simulink model "Cognata_Amp_Tobi_Split"  (R2020a)
settings: Solver=VariableStepAuto  StartTime=0.0  StopTime=inf  RelTol=1e-3
model workspace (MAT data in the model file):
  WinSize = Simulink.Parameter
  WinSize.Value = 16
  WinSize.DataType = 'double'
  WinSize.Dimensions = [1 1]
  fc_bandpass = Simulink.Parameter
  fc_bandpass.Value = [0.05 0.26]
  fc_bandpass.DataType = 'auto'
  fc_bandpass.Dimensions = [1 2]
undefined symbols (not defined in the file or in its folder): currentCFG_Cognata_Amp_Tobi_split_UB, fdesignblkfcn, gcbh, UB
libraries: gtecHighspeedLib x17, robotlib x12, dspfdesign x3, simulink x2, dsparch4 x2, TobiiEyeTrackerLib x1, gUSBamplib x1
settings Model: Creator=LAB-OREN3  LastModifiedBy=LAB-OREN3

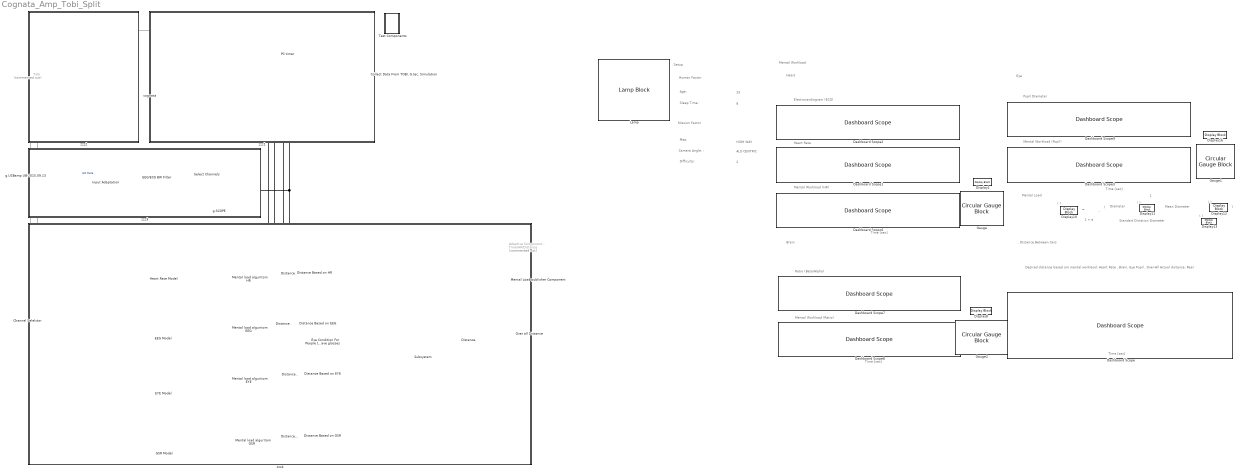
== system Cognata_Amp_Tobi_Split ==
  note: Time [sec]
  note: . Setup
  note: ( )
  note: Desired distance based om mental worklaod:
      | Heart Rate , Brain, Eye Pupil , Over-All
      |
      | Actual distance: Real
  note: Mission Factor
  note: Mental Workload (HR)
  note: Ratio (Beta/Alpha)
  note: 1
  note: Mental Load
  note: ( )
  note: Map:
  note: (
  note: HIGH WAY
  note: Mental Workload (Ratio)
  note: Eye
  note: 25
  note: Mean Diameter
  note: Time [sec]
  note: Diameter
  note: Human Factor
  note: Standart Diviation Diameter
  note: Age:
  note: Difficulty:
  note: 1 + e
  note: Camera Angle: :
  note: 8
  note: Sleep Time:
  note: Electrocardiogram (ECG)
  note: Heart
  note: Time [sec]
  note: ALO CENTRIC
  note: Brain
  note: Heart Rate
  note: ( )
  note: Pupil Diameter
  note: )
  note: -
  note: Mental Workload (Pupil)
  note: . Distance Between Cars
  note: 2
  note: ( )
  note: Time [sec]
  note: =
  note: Mental Workload
  "Adaptive Component - Time/HR/Distance " : Subsystem  Commented=on
  Channel Selelctor : Subsystem
  "Collect Data From TOBI, G.tec, Simulation" : Subsystem
  Dashboard Scope : DashboardScope  ShowInitialText=off  TimeSpan=10  Ymin=-1  Ymax=20  LegendPosition=Hide  ScaleAtStop=off
  Dashboard Scope1 : DashboardScope  TimeSpan=10  Ymin=0  Ymax=100  LegendPosition=Hide  ScaleAtStop=off
  Dashboard Scope2 : DashboardScope  TimeSpan=10  Ymin=-3000  Ymax=1000  LegendPosition=Hide  ScaleAtStop=off
  Dashboard Scope3 : DashboardScope  TimeSpan=10  Ymin=0  Ymax=1  LegendPosition=Hide  ScaleAtStop=off
  Dashboard Scope6 : DashboardScope  TimeSpan=10  Ymin=0  Ymax=1  LegendPosition=Hide  ScaleAtStop=off
  Dashboard Scope7 : DashboardScope  TimeSpan=10  Ymin=0  Ymax=0.5  LegendPosition=Hide  ScaleAtStop=off
  Dashboard Scope8 : DashboardScope  TimeSpan=10  Ymin=0  Ymax=1  LegendPosition=Hide  ScaleAtStop=off
  Dashboard Scope9 : DashboardScope  TimeSpan=10  Ymin=0  Ymax=5  LegendPosition=Hide  ScaleAtStop=off
  Display{1,8,10..11,13,16} (6 alike) : DisplayBlock  LabelPosition=Hide  Format=bank  Transparency=1
  Display12 : DisplayBlock  LabelPosition=Hide  Format=bank  Transparency=1  Layout=Fill available space
  Distance : MATLAB Function  TreatAsAtomicUnit=on
  Distance Based on EEG : Display
  Distance Based on EYE : Display
  Distance Based on GSR : Display
  Distance Based on HR : Display
  Distance, : MATLAB Function  TreatAsAtomicUnit=on
  Distance. : MATLAB Function  TreatAsAtomicUnit=on
  Distance.. : MATLAB Function  TreatAsAtomicUnit=on
  Distance... : MATLAB Function  TreatAsAtomicUnit=on
  EEG Model : Subsystem  ReferencedSubsystem=EEG_Ratio_Model
  EEG/ECG BW Filter : gtecHighspeedLib/EEG//ECG BW Filter  Order=6  LowerFreq=0.1  UpperFreq=30  SampFreq=512
      settings: SourceProductName=g.HIsys Library
  EYE Model : Subsystem  ReferencedSubsystem=Pupil_Diameter_Model
  Eye Condition For People that have glasses : Constant  Value=0
  GSR Model : Subsystem  ReferencedSubsystem=GSR_Model
  Gauge : CircularGaugeBlock  LabelPosition=Hide  ScaleMax=1  TickInterval=0.2
  Gauge1 : CircularGaugeBlock  LabelPosition=Hide  ScaleMax=1  TickInterval=0.2
  Gauge2 : CircularGaugeBlock  LabelPosition=Hide  ScaleMax=1  TickInterval=0.2
  Heart Rate Model : Subsystem  ReferencedSubsystem=Heart_Rate_Model
  Input Adaptation : Subsystem
  Lamp : LampBlock
  Mental Load publisher Component : Subsystem
  "Mental load alguritom EEG " : MATLAB Function  TreatAsAtomicUnit=on
  Mental load alguritom EYE : MATLAB Function  TreatAsAtomicUnit=on
  Mental load alguritom GSR : MATLAB Function  TreatAsAtomicUnit=on
  Mental load alguritom HR : MATLAB Function  TreatAsAtomicUnit=on
  Over all Distance : Display
  PC timer : MATLAB Function  TreatAsAtomicUnit=on
  Select Channels : gtecHighspeedLib/Select Channels  selectedchannels=[2]  totalchannels=14
      settings: SourceProductName=g.HIsys Library
  Subsystem : Subsystem
  Test Components : Subsystem
  Tobi : Subsystem  Commented=on
  cognata : Subsystem
  g.SCOPE : gtecHighspeedLib/g.SCOPE
      settings: SourceProductName=g.HIsys Library
  g.USBamp UB-2015.09.13 : gUSBamplib/g.USBamp  cfg=currentCFG_Cognata_Amp_Tobi_split_UB-2015.09.13.cfg  snr=UB-2015.09.13
      settings: SourceProductName=g.USBamp
  zzz1 : Subsystem  TreatAsAtomicUnit=on
      settings: OpenFcn=% no-op
      mask Display: disp('')
  zzz2 : Subsystem  TreatAsAtomicUnit=on
      settings: OpenFcn=% no-op
      mask Display: disp('')
  zzz3 : Subsystem  TreatAsAtomicUnit=on
      settings: OpenFcn=% no-op
      mask Display: disp('')
  zzz4 : Subsystem  TreatAsAtomicUnit=on
      settings: OpenFcn=% no-op
      mask Display: disp('')
  wires:
  cognata/3(Latitude) -> "Collect Data From TOBI, G.tec, Simulation"/6(Lat), "Adaptive Component - Time/HR/Distance "/3(Lat)
  Distance/1(y) -> Distance Based on HR/1
  EEG Model/1 -> "Mental load alguritom EEG "/1(u)
  Distance../1(y) -> Distance Based on EYE/1
  EYE Model/1 -> Mental load alguritom EYE/1(u)
  Distance,/1(y) -> Over all Distance/1
  g.USBamp UB-2015.09.13/1 -> Input Adaptation/1(In)  "EG Data"
  Mental load alguritom EYE/1(y) -> Distance../1(u), Subsystem/4(eye)
  Mental load alguritom HR/1(y) -> Subsystem/1(HR), Distance/1(u)
  Input Adaptation/1(All channels) -> Channel Selelctor/1(14x1 vec), "Collect Data From TOBI, G.tec, Simulation"/3(G.tec Channels), EEG/ECG BW Filter/1
  Distance./1(y) -> Distance Based on EEG/1
  Select Channels/1 -> ?
  cognata/4(TTC) -> "Collect Data From TOBI, G.tec, Simulation"/7(Distance)
  cognata/1(SimulationTime) -> "Adaptive Component - Time/HR/Distance "/1(Simlulation time), "Collect Data From TOBI, G.tec, Simulation"/4(Simulator time)
  EEG/ECG BW Filter/1 -> g.SCOPE/1, Select Channels/1
  cognata/2(Longitude) -> "Adaptive Component - Time/HR/Distance "/4(Long), "Collect Data From TOBI, G.tec, Simulation"/5(Long)
  "Mental load alguritom EEG "/1(y) -> Subsystem/2(Ratio), Distance./1(u)
  Heart Rate Model/2 -> Mental load alguritom HR/1(u)
  Tobi/1(Sum) -> "Collect Data From TOBI, G.tec, Simulation"/1(Tobi data)
  Mental load alguritom GSR/1(y) -> Distance.../1(u), Subsystem/5(GSR)
  GSR Model/1 -> Mental load alguritom GSR/1(u)
  Distance.../1(y) -> Distance Based on GSR/1
  Tobi/2(Pupil diameter Right) -> EYE Model/2
  Tobi/3("Pupil diameter Left ") -> EYE Model/1
  Subsystem/1(Avrage Mental Load) -> Distance,/1(u), "Adaptive Component - Time/HR/Distance "/2(Avrage Menta Load), Mental Load publisher Component/1(Mental Load)
  Eye Condition For People that have glasses/1 -> Subsystem/3(EyeCondition)
  Channel Selelctor/1(ECG) -> Heart Rate Model/1
  Channel Selelctor/2(EEG1) -> EEG Model/2
  Channel Selelctor/3(EEG2) -> EEG Model/3
  Channel Selelctor/4(EEG3) -> EEG Model/4
  Channel Selelctor/5(EEG4) -> EEG Model/5
  Channel Selelctor/6(EEG5) -> EEG Model/6
  Channel Selelctor/7(EEG6) -> EEG Model/7
  Channel Selelctor/8(EEG7) -> EEG Model/8
  Channel Selelctor/9(EEG8) -> EEG Model/9
  Channel Selelctor/10(EEG9) -> EEG Model/10
  Channel Selelctor/11(EEG10) -> EEG Model/11
  Channel Selelctor/12(EEG11) -> EEG Model/1
  Channel Selelctor/13(GSR) -> GSR Model/1
  PC timer/1(z) -> "Collect Data From TOBI, G.tec, Simulation"/2(PC timer)
  EYE Model/3 -> ?
  EYE Model/2 -> ?
  Channel Selelctor/14(EEG12) -> EEG Model/12

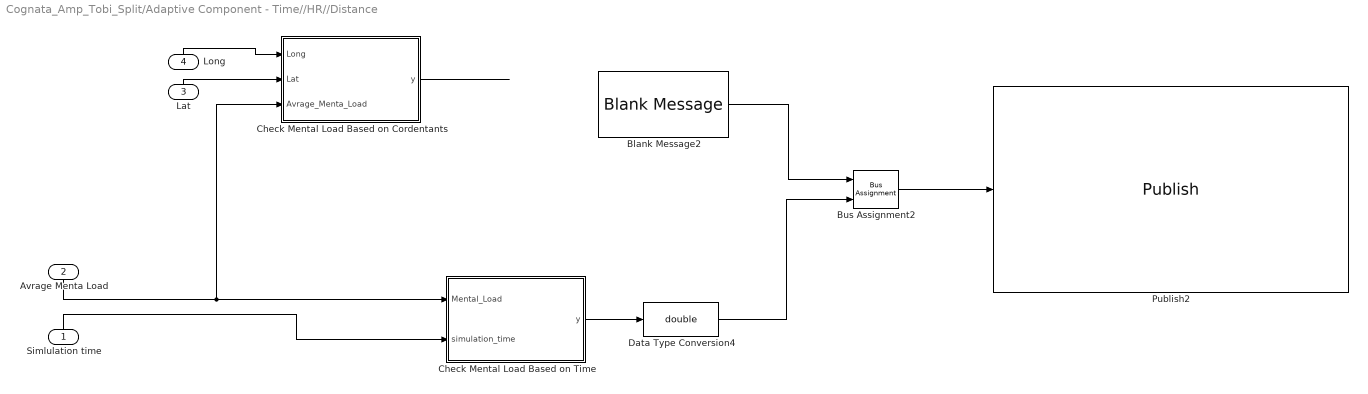
== system Cognata_Amp_Tobi_Split/Adaptive Component - Time//HR//Distance  ==
  Simlulation time : Inport
  Avrage Menta Load : Inport  Port=2
  Lat : Inport  Port=3
  Long : Inport  Port=4
  Blank Message2 : robotlib/Blank Message  messageClass=Message  entityType=std_msgs/Float64  messageType=std_msgs/Float64  SampleTime=inf
  Bus Assignment2 : BusAssignment  AssignedSignals=Data
  Check Mental Load Based on Cordentants : MATLAB Function  TreatAsAtomicUnit=on
  Check Mental Load Based on Time : MATLAB Function  TreatAsAtomicUnit=on
  Data Type Conversion4 : DataTypeConversion  OutDataTypeStr=double
  Publish2 : robotlib/Publish  topicSource=Specify your own  topic=/Test1  messageType=std_msgs/Float64  messageQueueLength=1
  wires:
  Check Mental Load Based on Time/1(y) -> Data Type Conversion4/1
  Simlulation time/1 -> Check Mental Load Based on Time/2(simulation_time)
  Avrage Menta Load/1 -> Check Mental Load Based on Cordentants/3(Avrage_Menta_Load), Check Mental Load Based on Time/1(Mental_Load)
  Bus Assignment2/1 -> Publish2/1
  Blank Message2/1 -> Bus Assignment2/1
  Data Type Conversion4/1 -> Bus Assignment2/2
  Long/1 -> Check Mental Load Based on Cordentants/1(Long)
  Lat/1 -> Check Mental Load Based on Cordentants/2(Lat)
  Check Mental Load Based on Cordentants/1(y) -> ?

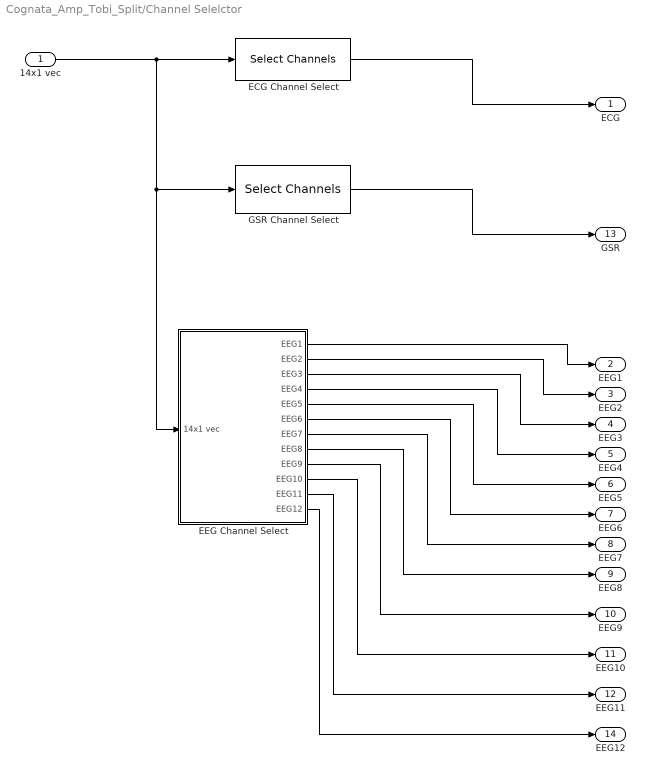
== system Cognata_Amp_Tobi_Split/Channel Selelctor ==
  14x1 vec : Inport
  ECG Channel Select : gtecHighspeedLib/Select Channels  selectedchannels=[2]  totalchannels=14
      settings: SourceProductName=g.HIsys Library
  EEG Channel Select : Subsystem
  GSR Channel Select : gtecHighspeedLib/Select Channels  selectedchannels=[1]  totalchannels=14
      settings: SourceProductName=g.HIsys Library
  ECG : Outport
  EEG1 : Outport  Port=2
  EEG2 : Outport  Port=3
  EEG3 : Outport  Port=4
  EEG4 : Outport  Port=5
  EEG5 : Outport  Port=6
  EEG6 : Outport  Port=7
  EEG7 : Outport  Port=8
  EEG8 : Outport  Port=9
  EEG9 : Outport  Port=10
  EEG10 : Outport  Port=11
  EEG11 : Outport  Port=12
  GSR : Outport  Port=13
  EEG12 : Outport  Port=14
  wires:
  14x1 vec/1 -> ECG Channel Select/1, GSR Channel Select/1, EEG Channel Select/1(14x1 vec)
  ECG Channel Select/1 -> ECG/1
  GSR Channel Select/1 -> GSR/1
  EEG Channel Select/1(EEG1) -> EEG1/1
  EEG Channel Select/2(EEG2) -> EEG2/1
  EEG Channel Select/3(EEG3) -> EEG3/1
  EEG Channel Select/4(EEG4) -> EEG4/1
  EEG Channel Select/5(EEG5) -> EEG5/1
  EEG Channel Select/6(EEG6) -> EEG6/1
  EEG Channel Select/7(EEG7) -> EEG7/1
  EEG Channel Select/8(EEG8) -> EEG8/1
  EEG Channel Select/9(EEG9) -> EEG9/1
  EEG Channel Select/10(EEG10) -> EEG10/1
  EEG Channel Select/11(EEG11) -> EEG11/1
  EEG Channel Select/12(EEG12) -> EEG12/1

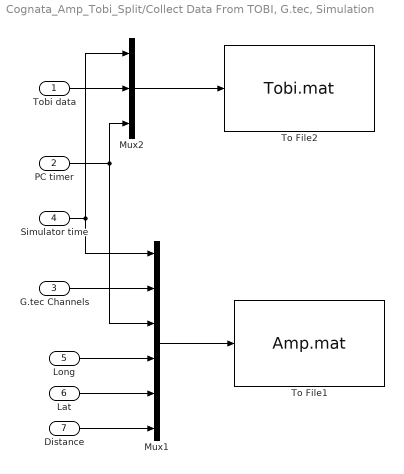
== system Cognata_Amp_Tobi_Split/Collect Data From TOBI, G.tec, Simulation ==
  Tobi data : Inport
  PC timer : Inport  Port=2
  G.tec Channels : Inport  Port=3
  Simulator time : Inport  Port=4
  Long : Inport  Port=5
  Lat : Inport  Port=6
  Distance : Inport  Port=7
  Mux1 : Mux  Inputs=6
  Mux2 : Mux  Inputs=3
  To File1 : ToFile  Filename=Amp.mat  MatrixName=Ampdata
  To File2 : ToFile  Filename=Tobi.mat  MatrixName=Tobidata
  wires:
  Tobi data/1 -> Mux2/2
  Simulator time/1 -> Mux1/1, Mux2/1
  Mux1/1 -> To File1/1
  Mux2/1 -> To File2/1
  Long/1 -> Mux1/4
  Distance/1 -> Mux1/6
  G.tec Channels/1 -> Mux1/2
  Lat/1 -> Mux1/5
  PC timer/1 -> Mux1/3, Mux2/3

== system Cognata_Amp_Tobi_Split/Input Adaptation ==
  In : Inport
  Data Type Conversion : DataTypeConversion  OutDataTypeStr=double
  Unbuffer : Unbuffer
  All channels : Outport
  wires:
  In/1 -> Unbuffer/1
  Unbuffer/1 -> Data Type Conversion/1
  Data Type Conversion/1 -> All channels/1

== system Cognata_Amp_Tobi_Split/Mental Load publisher Component ==
  Mental Load : Inport
  Blank Message2 : robotlib/Blank Message  messageClass=Message  entityType=std_msgs/Float64  messageType=std_msgs/Float64  SampleTime=0
  Bus Assignment2 : BusAssignment  AssignedSignals=Data
  Publish : robotlib/Publish  topicSource=Specify your own  topic=/HR  messageType=std_msgs/Float64  messageQueueLength=1
  wires:
  Mental Load/1 -> Bus Assignment2/2
  Blank Message2/1 -> Bus Assignment2/1
  Bus Assignment2/1 -> Publish/1

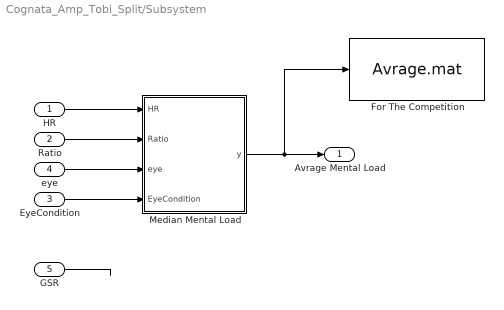
== system Cognata_Amp_Tobi_Split/Subsystem ==
  HR : Inport
  Ratio : Inport  Port=2
  EyeCondition : Inport  Port=3
  eye : Inport  Port=4
  GSR : Inport  Port=5
  For The Competition : ToFile  Filename=Avrage.mat  MatrixName=Avrage
  Median Mental Load : MATLAB Function  TreatAsAtomicUnit=on
  Avrage Mental Load : Outport
  wires:
  EyeCondition/1 -> Median Mental Load/4(EyeCondition)
  Median Mental Load/1(y) -> For The Competition/1, Avrage Mental Load/1
  Ratio/1 -> Median Mental Load/2(Ratio)
  eye/1 -> Median Mental Load/3(eye)
  HR/1 -> Median Mental Load/1(HR)
  GSR/1 -> ?

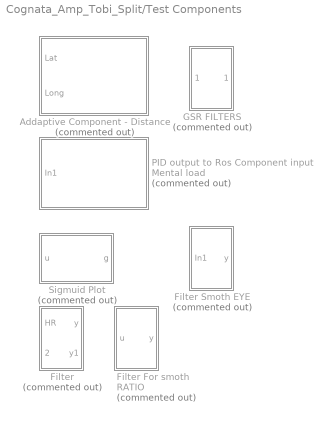
== system Cognata_Amp_Tobi_Split/Test Components ==
  Addaptive Component - Distance : Subsystem  Commented=on
  Filter : Subsystem  Commented=on
  Filter For smoth RATIO : Subsystem  Commented=on
  Filter Smoth EYE : Subsystem  Commented=on
  GSR FILTERS : Subsystem  Commented=on
  PID output to Ros Component input Mental load : Subsystem  Commented=on
  Sigmuid Plot : MATLAB Function  Commented=on  TreatAsAtomicUnit=on

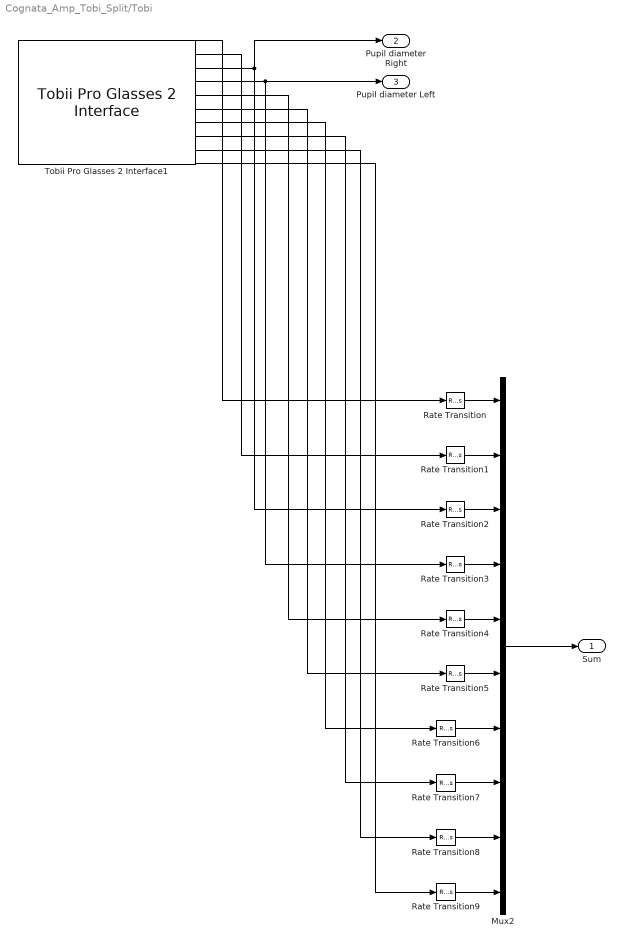
== system Cognata_Amp_Tobi_Split/Tobi ==
  Mux2 : Mux  Inputs=10
  Rate Transition{,1..9} (10 alike) : RateTransition  Deterministic=off  OutPortSampleTimeOpt=Inherit
  Tobii Pro Glasses 2 Interface1 : TobiiEyeTrackerLib/Tobii Pro Glasses 2 Interface  Key=0  pc_right=off  pc_left=off  pd_right=off  pd_left=off  gd_right=off  gd_left=off  gp=on  gp3=off  gy=off  ac=off
      settings: SourceProductName=g.EYEtracking Interface (Tobii Pro Glasses 2)
  Sum : Outport
  Pupil diameter Right : Outport  Port=2
  "Pupil diameter Left " : Outport  Port=3
  wires:
  Rate Transition2/1 -> Mux2/3
  Rate Transition6/1 -> Mux2/7
  Tobii Pro Glasses 2 Interface1/4 -> "Pupil diameter Left "/1, Rate Transition3/1
  Tobii Pro Glasses 2 Interface1/1 -> Rate Transition/1
  Rate Transition1/1 -> Mux2/2
  Mux2/1 -> Sum/1
  Tobii Pro Glasses 2 Interface1/3 -> Pupil diameter Right/1, Rate Transition2/1
  Tobii Pro Glasses 2 Interface1/8 -> Rate Transition7/1
  Tobii Pro Glasses 2 Interface1/5 -> Rate Transition4/1
  Tobii Pro Glasses 2 Interface1/10 -> Rate Transition9/1
  Tobii Pro Glasses 2 Interface1/2 -> Rate Transition1/1
  Tobii Pro Glasses 2 Interface1/9 -> Rate Transition8/1
  Tobii Pro Glasses 2 Interface1/7 -> Rate Transition6/1
  Rate Transition/1 -> Mux2/1
  Rate Transition4/1 -> Mux2/5
  Tobii Pro Glasses 2 Interface1/6 -> Rate Transition5/1
  Rate Transition5/1 -> Mux2/6
  Rate Transition3/1 -> Mux2/4
  Rate Transition8/1 -> Mux2/9
  Rate Transition9/1 -> Mux2/10
  Rate Transition7/1 -> Mux2/8

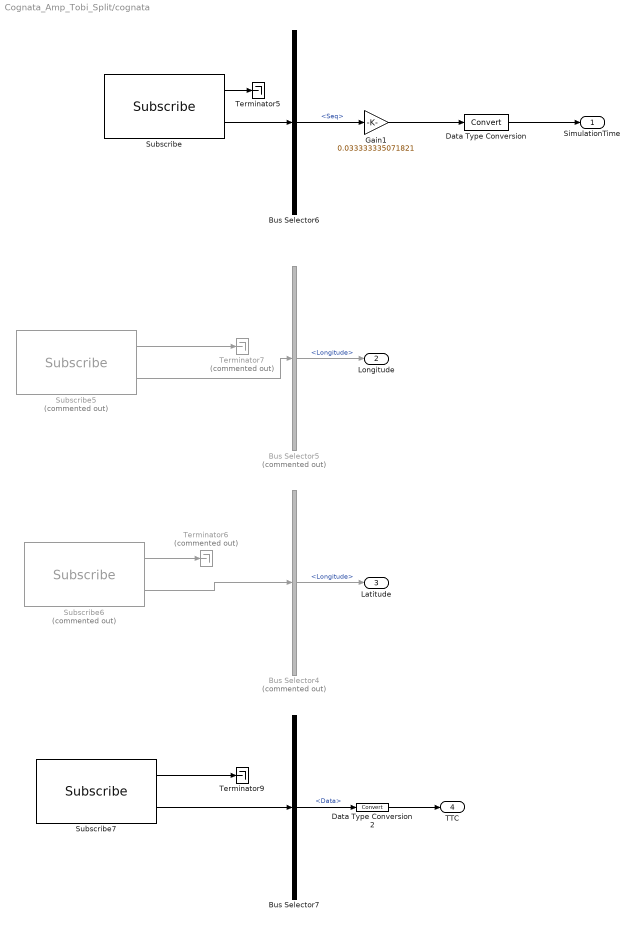
== system Cognata_Amp_Tobi_Split/cognata ==
  Bus Selector4 : BusSelector  Commented=on  OutputSignals=Longitude
  Bus Selector5 : BusSelector  Commented=on  OutputSignals=Longitude
  Bus Selector6 : BusSelector  OutputSignals=Header.Seq
  Bus Selector7 : BusSelector  OutputSignals=Data
  Data Type Conversion : DataTypeConversion
  Data Type Conversion2 : DataTypeConversion
  Gain1 : Gain  Gain=0.033333335071821
  Subscribe : robotlib/Subscribe  topicSource=Specify your own  topic=/cognataSDK/GPS/info  messageType=sensor_msgs/NavSatFix  sampleTime=0.5  messageQueueLength=1
  Subscribe5 : robotlib/Subscribe  Commented=on  topicSource=Specify your own  topic=/cognataSDK/GPS/info  messageType=sensor_msgs/NavSatFix  sampleTime=-1  messageQueueLength=1
  Subscribe6 : robotlib/Subscribe  Commented=on  topicSource=Specify your own  topic=/cognataSDK/GPS/info  messageType=sensor_msgs/NavSatFix  sampleTime=-1  messageQueueLength=1
  Subscribe7 : robotlib/Subscribe  topicSource=Specify your own  topic=/Distance_topic  messageType=std_msgs/Float32  sampleTime=0.5  messageQueueLength=1
  Terminator5 : Terminator
  Terminator6 : Terminator  Commented=on
  Terminator7 : Terminator  Commented=on
  Terminator9 : Terminator
  SimulationTime : Outport
  Longitude : Outport  Port=2
  Latitude : Outport  Port=3
  TTC : Outport  Port=4
  wires:
  Subscribe/1 -> Terminator5/1
  Bus Selector4/1 -> Latitude/1  "<Longitude>"
  Subscribe6/2 -> Bus Selector4/1
  Subscribe6/1 -> Terminator6/1
  Bus Selector5/1 -> Longitude/1  "<Longitude>"
  Subscribe5/2 -> Bus Selector5/1
  Subscribe5/1 -> Terminator7/1
  Subscribe/2 -> Bus Selector6/1
  Bus Selector6/1 -> Gain1/1  "<Seq>"
  Subscribe7/2 -> Bus Selector7/1
  Subscribe7/1 -> Terminator9/1
  Bus Selector7/1 -> Data Type Conversion2/1  "<Data>"
  Gain1/1 -> Data Type Conversion/1
  Data Type Conversion/1 -> SimulationTime/1
  Data Type Conversion2/1 -> TTC/1

== system Cognata_Amp_Tobi_Split/zzz1 ==

== system Cognata_Amp_Tobi_Split/zzz2 ==

== system Cognata_Amp_Tobi_Split/zzz3 ==

== system Cognata_Amp_Tobi_Split/zzz4 ==

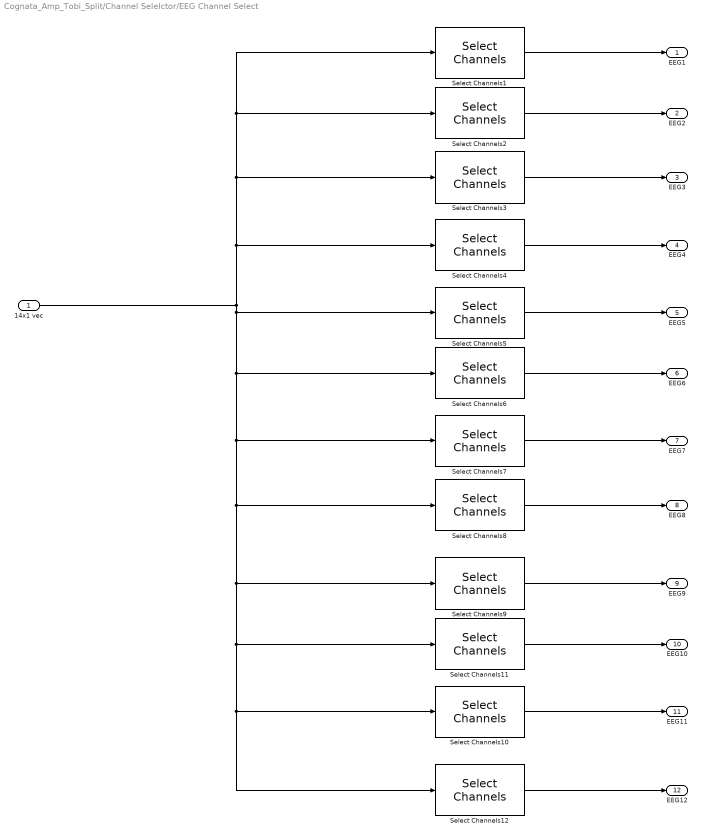
== system Cognata_Amp_Tobi_Split/Channel Selelctor/EEG Channel Select ==
  14x1 vec : Inport
  Select Channels1 : gtecHighspeedLib/Select Channels  selectedchannels=[3]  totalchannels=14
      settings: SourceProductName=g.HIsys Library
  Select Channels10 : gtecHighspeedLib/Select Channels  selectedchannels=[13]  totalchannels=14
      settings: SourceProductName=g.HIsys Library
  Select Channels11 : gtecHighspeedLib/Select Channels  selectedchannels=[12]  totalchannels=14
      settings: SourceProductName=g.HIsys Library
  Select Channels12 : gtecHighspeedLib/Select Channels  selectedchannels=[13]  totalchannels=14
      settings: SourceProductName=g.HIsys Library
  Select Channels2 : gtecHighspeedLib/Select Channels  selectedchannels=[4]  totalchannels=14
      settings: SourceProductName=g.HIsys Library
  Select Channels3 : gtecHighspeedLib/Select Channels  selectedchannels=[5]  totalchannels=14
      settings: SourceProductName=g.HIsys Library
  Select Channels4 : gtecHighspeedLib/Select Channels  selectedchannels=[6]  totalchannels=14
      settings: SourceProductName=g.HIsys Library
  Select Channels5 : gtecHighspeedLib/Select Channels  selectedchannels=[7]  totalchannels=14
      settings: SourceProductName=g.HIsys Library
  Select Channels6 : gtecHighspeedLib/Select Channels  selectedchannels=[8]  totalchannels=14
      settings: SourceProductName=g.HIsys Library
  Select Channels7 : gtecHighspeedLib/Select Channels  selectedchannels=[9]  totalchannels=14
      settings: SourceProductName=g.HIsys Library
  Select Channels8 : gtecHighspeedLib/Select Channels  selectedchannels=[10]  totalchannels=14
      settings: SourceProductName=g.HIsys Library
  Select Channels9 : gtecHighspeedLib/Select Channels  selectedchannels=[11]  totalchannels=14
      settings: SourceProductName=g.HIsys Library
  EEG1 : Outport
  EEG2 : Outport  Port=2
  EEG3 : Outport  Port=3
  EEG4 : Outport  Port=4
  EEG5 : Outport  Port=5
  EEG6 : Outport  Port=6
  EEG7 : Outport  Port=7
  EEG8 : Outport  Port=8
  EEG9 : Outport  Port=9
  EEG10 : Outport  Port=10
  EEG11 : Outport  Port=11
  EEG12 : Outport  Port=12
  wires:
  Select Channels7/1 -> EEG7/1
  Select Channels1/1 -> EEG1/1
  Select Channels8/1 -> EEG8/1
  Select Channels11/1 -> EEG10/1
  Select Channels2/1 -> EEG2/1
  Select Channels4/1 -> EEG4/1
  Select Channels5/1 -> EEG5/1
  Select Channels10/1 -> EEG11/1
  Select Channels9/1 -> EEG9/1
  Select Channels6/1 -> EEG6/1
  Select Channels3/1 -> EEG3/1
  14x1 vec/1 -> Select Channels8/1, Select Channels10/1, Select Channels12/1, Select Channels11/1, Select Channels9/1, Select Channels7/1, Select Channels6/1, Select Channels5/1, Select Channels4/1, Select Channels2/1, Select Channels1/1, Select Channels3/1
  Select Channels12/1 -> EEG12/1

== system Cognata_Amp_Tobi_Split/Test Components/Addaptive Component - Distance ==
  Lat : Inport
  Long : Inport  Port=2
  Blank Message2 : robotlib/Blank Message  SourceLibraryInfo=This block requires Robotics System Toolbox  messageType=std_msgs/Float64  SampleTime=inf
  Bus Assignment2 : BusAssignment  AssignedSignals=Data
  Data Type Conversion4 : DataTypeConversion  OutDataTypeStr=double
  MATLAB Function : MATLAB Function  TreatAsAtomicUnit=on
  Publish2 : robotlib/Publish  SourceLibraryInfo=This block requires Robotics System Toolbox  topicSource=Specify your own  topic=/Test1  messageType=std_msgs/Float64  messageQueueLength=1
  wires:
  MATLAB Function/1(y) -> Data Type Conversion4/1
  Lat/1 -> MATLAB Function/2(Lat1)
  Bus Assignment2/1 -> Publish2/1
  Blank Message2/1 -> Bus Assignment2/1
  Data Type Conversion4/1 -> Bus Assignment2/2
  Long/1 -> ?

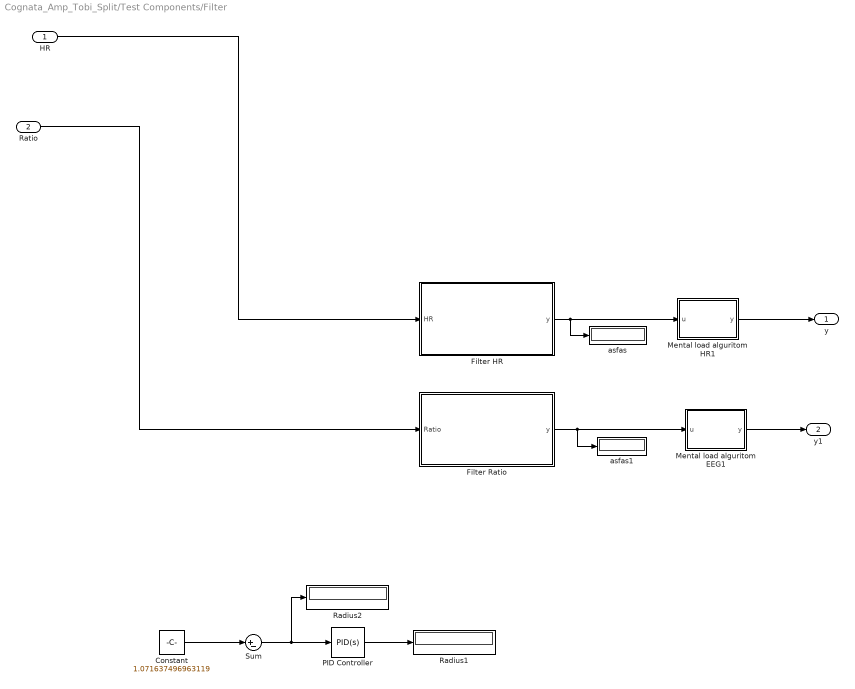
== system Cognata_Amp_Tobi_Split/Test Components/Filter ==
  HR : Inport
  Ratio : Inport  Port=2
  Constant : Constant  Value=1.071637496963119
  Filter HR : MATLAB Function  TreatAsAtomicUnit=on
  Filter Ratio : MATLAB Function  TreatAsAtomicUnit=on
  Mental load alguritom EEG1 : MATLAB Function  TreatAsAtomicUnit=on
  Mental load alguritom HR1 : MATLAB Function  TreatAsAtomicUnit=on
  PID Controller : simulink/Continuous/PID Controller  Controller=PID  Form=Parallel  TimeDomain=Continuous-time  UseExternalTs=off  SampleTime=-1  IntegratorMethod=Forward Euler  FilterMethod=Forward Euler  ControllerParametersSource=internal  P=0  I=5  D=0  UseFilter=on  N=100  TunerSelectOption=Transfer Function Based (PID Tuner App)  InitialConditionSource=internal  InitialConditionForIntegrator=0  InitialConditionForFilter=0  DifferentiatorICPrevScaledInput=0  ExternalReset=none  TrackingMode=off  Kt=1  LimitOutput=off  UpperSaturationLimit=inf  LowerSaturationLimit=-inf  LinearizeAsGain=on  AntiWindupMode=none  Kb=1  POutMin=[]  POutMax=[]  IOutMin=[]  IOutMax=[]  DOutMin=[]  DOutMax=[]  NOutMin=[]  NOutMax=[]  SumOutMin=[]  SumOutMax=[]  SaturationOutMin=[]  SaturationOutMax=[]  PParamMin=[]  PParamMax=[]  IParamMin=[]  IParamMax=[]  DParamMin=[]  DParamMax=[]  NParamMin=[]  NParamMax=[]  KbParamMin=[]  KbParamMax=[]  KtParamMin=[]  KtParamMax=[]  KbOutMin=[]  KbOutMax=[]  KtOutMin=[]  KtOutMax=[]  IntegratorOutMin=[]  IntegratorOutMax=[]  FilterOutMin=[]  FilterOutMax=[]  SumI1OutMin=[]  SumI1OutMax=[]  SumI2OutMin=[]  SumI2OutMax=[]  SumI3OutMin=[]  SumI3OutMax=[]  SumI4OutMin=[]  SumI4OutMax=[]  SumDOutMin=[]  SumDOutMax=[]  DifferentiatorOutMin=[]  DifferentiatorOutMax=[]  FilterDiffOutCoefMin=[]  FilterDiffOutCoefMax=[]  ReciprocalOutMin=[]  ReciprocalOutMax=[]  SumDenOutMin=[]  SumDenOutMax=[]  SumNumOutMin=[]  SumNumOutMax=[]  DivideOutMin=[]  DivideOutMax=[]  UdiffTsProdOutMin=[]  UdiffTsProdOutMax=[]  NTsProdOutMin=[]  NTsProdOutMax=[]  UintegralTsProdOutMin=[]  UintegralTsProdOutMax=[]  UngainTsProdOutMin=[]  UngainTsProdOutMax=[]  IntegratorContinuousStateAttributes=''  IntegratorStateMustResolveToSignalObject=off  IntegratorRTWStateStorageClass=Auto  FilterContinuousStateAttributes=''  FilterStateMustResolveToSignalObject=off  FilterRTWStateStorageClass=Auto  ParallelPVariant=InternalParameters  IdealPVariant=Disabled  IVariant=InternalParameters  DVariant=InternalParameters  IntegratorVariant=Continuous  SatVariant=Disabled  AWVariant=Passthrough  PCopyVariant=Disabled  TRVariant=Disabled  FdbkBlocksVariant=Forward  IdealPFdbkVariant=Disabled  SatFdbkVariant=Disabled  DerivativeFilterVariant=ContFilter  NVariant=InternalParameters  NCopyVariant=Disabled  FilterICVariant=InternalICsFilter  IntegratorICVariant=InternalICs  ExternalResetVariant=Disabled  TRSumVariant=Passthrough  SumFdbkVariant=Disabled  SumVariant=Sum_PID  TsampFilterVariant=InternalTs  TsampNgainVariant=Passthrough  TsampIntegralVariant=Passthrough
  Radius1 : Display
  Radius2 : Display
  Sum : Sum  Inputs=|+-
  asfas : Display
  asfas1 : Display
  y : Outport
  y1 : Outport  Port=2
  wires:
  Filter Ratio/1(y) -> Mental load alguritom EEG1/1(u), asfas1/1
  Filter HR/1(y) -> Mental load alguritom HR1/1(u), asfas/1
  Mental load alguritom EEG1/1(y) -> y1/1
  HR/1 -> Filter HR/1(HR)
  Ratio/1 -> Filter Ratio/1(Ratio)
  Mental load alguritom HR1/1(y) -> y/1
  Constant/1 -> Sum/1
  Sum/1 -> Radius2/1, PID Controller/1
  PID Controller/1 -> Radius1/1
  ? -> Sum/2

== system Cognata_Amp_Tobi_Split/Test Components/Filter For smoth RATIO ==
  u : Inport
  MATLAB Function2 : MATLAB Function  TreatAsAtomicUnit=on
  MATLAB Function4 : MATLAB Function  TreatAsAtomicUnit=on
  Mental load alguritom EEG1 : MATLAB Function  TreatAsAtomicUnit=on
  Radius3 : Display
  Transfer Fcn : TransferFcn  Numerator=1  Denominator=[1 1]
  y : Outport
  wires:
  Transfer Fcn/1 -> Mental load alguritom EEG1/1(u), Radius3/1
  MATLAB Function2/1(y) -> Transfer Fcn/1
  Mental load alguritom EEG1/1(y) -> MATLAB Function4/1(u)
  u/1 -> MATLAB Function2/1(u)
  MATLAB Function4/1(y) -> y/1

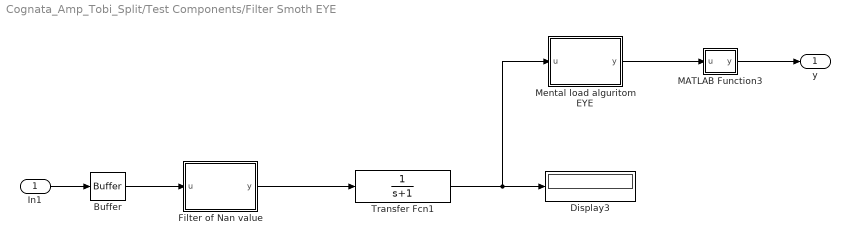
== system Cognata_Amp_Tobi_Split/Test Components/Filter Smoth EYE ==
  In1 : Inport
  Buffer : Buffer  N=30  OutputFrames=off
  Display3 : Display
  Filter of Nan value : MATLAB Function  TreatAsAtomicUnit=on
  MATLAB Function3 : MATLAB Function  TreatAsAtomicUnit=on
  Mental load alguritom EYE : MATLAB Function  TreatAsAtomicUnit=on
  Transfer Fcn1 : TransferFcn  Numerator=1  Denominator=[1 1]
  y : Outport
  wires:
  Buffer/1 -> Filter of Nan value/1(u)
  Filter of Nan value/1(y) -> Transfer Fcn1/1
  Transfer Fcn1/1 -> Mental load alguritom EYE/1(u), Display3/1
  Mental load alguritom EYE/1(y) -> MATLAB Function3/1(u)
  MATLAB Function3/1(y) -> y/1
  In1/1 -> Buffer/1

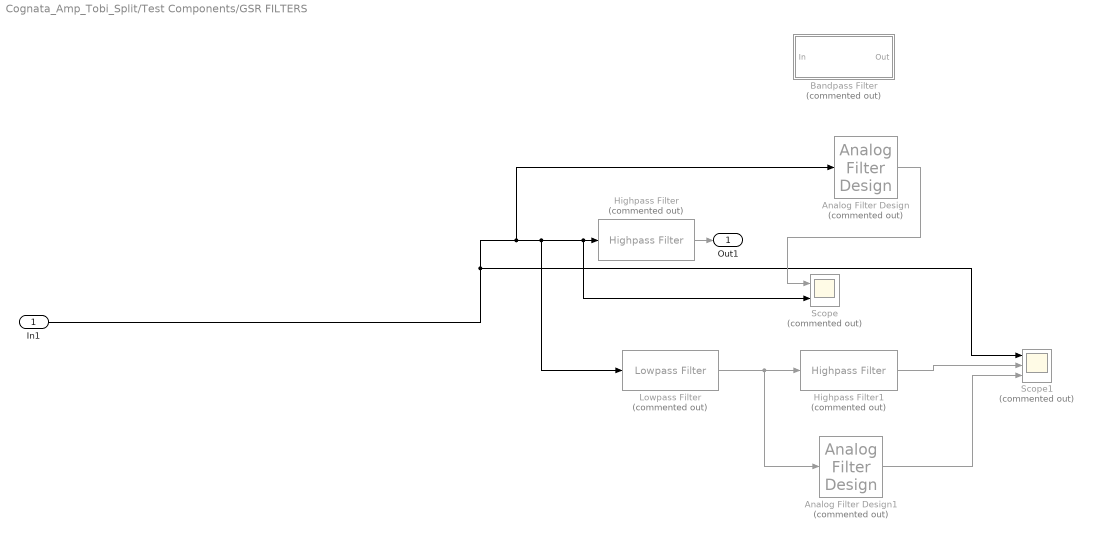
== system Cognata_Amp_Tobi_Split/Test Components/GSR FILTERS ==
  In1 : Inport
  Analog Filter Design : dsparch4/Analog Filter Design  Commented=on  method=Butterworth  filttype=Highpass  N=8  Wlo=0.05  Whi=80  Rp=2  Rs=40
  Analog Filter Design1 : dsparch4/Analog Filter Design  Commented=on  method=Butterworth  filttype=Highpass  N=50  Wlo=0.0001953125  Whi=80  Rp=2  Rs=40
  Bandpass Filter : Subsystem  Commented=on  DialogController=fdesignblkfcn  InitFcn=fdesignblkfcn(gcbh, {'InitFcn'});  mask(Bandpass Filter){}
      mask help: Design a bandpass filter
      settings: CopyFcn=fdesignblkfcn(gcbh, {'CopyFcn'});
      mask Help: helpview(mapfilelocation('dsp'), 'dspbandpassfilter');
      mask Display: disp('Bandpass');
  Highpass Filter : dspfdesign/Highpass Filter  Commented=on  FilterType=FIR  DesignForMinimumOrder=off  FilterOrder=50  StopbandFrequency=0.05  PassbandFrequency=0.05  StopbandAttenuation=80  PassbandRipple=0.1  InheritSampleRate=off  SampleRate=512  SimulateUsing=Interpreted execution  roundingMode=Floor  coeffsDataTypeStr=fixdt(1,16)
  Highpass Filter1 : dspfdesign/Highpass Filter  Commented=on  FilterType=FIR  DesignForMinimumOrder=off  FilterOrder=50  StopbandFrequency=8e3  PassbandFrequency=1  StopbandAttenuation=80  PassbandRipple=0.1  InheritSampleRate=on  SampleRate=512  SimulateUsing=Interpreted execution  roundingMode=Floor  coeffsDataTypeStr=fixdt(1,16)
  Lowpass Filter : dspfdesign/Lowpass Filter  Commented=on  FilterType=FIR  DesignForMinimumOrder=off  FilterOrder=50  PassbandFrequency=5  StopbandFrequency=12e3  PassbandRipple=0.1  StopbandAttenuation=80  InheritSampleRate=on  SampleRate=512  SimulateUsing=Interpreted execution  roundingMode=Floor  coeffsDataTypeStr=fixdt(1,16)
  Scope : Scope  Commented=on  NumInputPorts=2
  Scope1 : Scope  Commented=on  NumInputPorts=3
  Out1 : Outport
  wires:
  Lowpass Filter/1 -> Analog Filter Design1/1, Highpass Filter1/1
  In1/1 -> Analog Filter Design/1, Lowpass Filter/1, Scope/2, Highpass Filter/1, Scope1/1
  Highpass Filter/1 -> Out1/1
  Analog Filter Design1/1 -> Scope1/3
  Analog Filter Design/1 -> Scope/1
  Highpass Filter1/1 -> Scope1/2

== system Cognata_Amp_Tobi_Split/Test Components/PID output to Ros Component input Mental load ==
  In1 : Inport
  Constant : Constant
  PID Controller : simulink/Continuous/PID Controller  Controller=PID  Form=Parallel  TimeDomain=Continuous-time  UseExternalTs=off  SampleTime=-1  IntegratorMethod=Forward Euler  FilterMethod=Forward Euler  ControllerParametersSource=internal  P=1  I=1  D=0  UseFilter=on  N=100  TunerSelectOption=Transfer Function Based (PID Tuner App)  InitialConditionSource=internal  InitialConditionForIntegrator=0  InitialConditionForFilter=0  DifferentiatorICPrevScaledInput=0  ExternalReset=none  TrackingMode=off  Kt=1  LimitOutput=off  UpperSaturationLimit=inf  LowerSaturationLimit=-inf  LinearizeAsGain=on  AntiWindupMode=none  Kb=1  POutMin=[]  POutMax=[]  IOutMin=[]  IOutMax=[]  DOutMin=[]  DOutMax=[]  NOutMin=[]  NOutMax=[]  SumOutMin=[]  SumOutMax=[]  SaturationOutMin=[]  SaturationOutMax=[]  PParamMin=[]  PParamMax=[]  IParamMin=[]  IParamMax=[]  DParamMin=[]  DParamMax=[]  NParamMin=[]  NParamMax=[]  KbParamMin=[]  KbParamMax=[]  KtParamMin=[]  KtParamMax=[]  KbOutMin=[]  KbOutMax=[]  KtOutMin=[]  KtOutMax=[]  IntegratorOutMin=[]  IntegratorOutMax=[]  FilterOutMin=[]  FilterOutMax=[]  SumI1OutMin=[]  SumI1OutMax=[]  SumI2OutMin=[]  SumI2OutMax=[]  SumI3OutMin=[]  SumI3OutMax=[]  SumI4OutMin=[]  SumI4OutMax=[]  SumDOutMin=[]  SumDOutMax=[]  DifferentiatorOutMin=[]  DifferentiatorOutMax=[]  FilterDiffOutCoefMin=[]  FilterDiffOutCoefMax=[]  ReciprocalOutMin=[]  ReciprocalOutMax=[]  SumDenOutMin=[]  SumDenOutMax=[]  SumNumOutMin=[]  SumNumOutMax=[]  DivideOutMin=[]  DivideOutMax=[]  UdiffTsProdOutMin=[]  UdiffTsProdOutMax=[]  NTsProdOutMin=[]  NTsProdOutMax=[]  UintegralTsProdOutMin=[]  UintegralTsProdOutMax=[]  UngainTsProdOutMin=[]  UngainTsProdOutMax=[]  IntegratorContinuousStateAttributes=''  IntegratorStateMustResolveToSignalObject=off  IntegratorRTWStateStorageClass=Auto  FilterContinuousStateAttributes=''  FilterStateMustResolveToSignalObject=off  FilterRTWStateStorageClass=Auto  ParallelPVariant=InternalParameters  IdealPVariant=Disabled  IVariant=InternalParameters  DVariant=InternalParameters  IntegratorVariant=Continuous  SatVariant=Disabled  AWVariant=Passthrough  PCopyVariant=Disabled  TRVariant=Disabled  FdbkBlocksVariant=Forward  IdealPFdbkVariant=Disabled  SatFdbkVariant=Disabled  DerivativeFilterVariant=ContFilter  NVariant=InternalParameters  NCopyVariant=Disabled  FilterICVariant=InternalICsFilter  IntegratorICVariant=InternalICs  ExternalResetVariant=Disabled  TRSumVariant=Passthrough  SumFdbkVariant=Disabled  SumVariant=Sum_PID  TsampFilterVariant=InternalTs  TsampNgainVariant=Passthrough  TsampIntegralVariant=Passthrough
  Ros Component1 : Subsystem
  Sum : Sum  Inputs=+-
  wires:
  Sum/1 -> PID Controller/1
  Constant/1 -> Sum/1
  PID Controller/1 -> Ros Component1/1(In1)
  In1/1 -> Sum/2

== system Cognata_Amp_Tobi_Split/Test Components/GSR FILTERS/Bandpass Filter ==
  In : Inport
  Generated Filter Block : DiscreteFir  Tag=BlockMethodSubSystem  Coefficients=[-0.0008992291487744296 0.0016414518747943749 0.0031352071842225397 -0.0040707550828814922 -0.0063731852227904111 0.0074874286806090491 0.0098354319566295711 -0.010189316513446216 -0.011302794465874122 0.0096929185841818435 0.0079428653987464216 -0.0031368247881221642 0.0028299878877943137 -0.011508674243001471 -0.022080136219461581 0.034245325424507672 0.048356661648905473 -0.062355369169884239 -0.077503478162593897 0.090687768153125653 0.10353171105844157 -0.11297860084229834 -0.12035866024978455 0.12379360801539134 0.12379360801539134 -0.12035866024978455 -0.11297860084229834 0.10353171105844157 0.090687768153125653 -0.077503478162593897 -0.062355369169884239 0.048356661648905473 0.034245325424507672 -0.022080136219461581 -0.011508674243001471 0.0028299878877943137 -0.0031368247881221642 0.0079428653987464216 0.0096929185841818435 -0.011302794465874122 -0.010189316513446216 0.0098354319566295711 0.0074874286806090491 -0.0063731852227904111 -0.0040707550828814922 0.0031352071842225397 0.0016414518747943749 -0.0008992291487744296]  InputProcessing=Columns as channels (frame based)
  Out : Outport  VectorParamsAs1DForOutWhenUnconnected=off
  wires:
  In/1 -> Generated Filter Block/1
  Generated Filter Block/1 -> Out/1

== system Cognata_Amp_Tobi_Split/Test Components/PID output to Ros Component input Mental load/Ros Component1 ==
  In1 : Inport
  Blank Message1 : robotlib/Blank Message  SourceLibraryInfo=This block requires Robotics System Toolbox  messageType=std_msgs/Float64  SampleTime=inf
  Bus Assignment1 : BusAssignment  AssignedSignals=Data
  Display1 : Display
  Publish1 : robotlib/Publish  SourceLibraryInfo=This block requires Robotics System Toolbox  topicSource=Specify your own  topic=/HR  messageType=std_msgs/Float64  messageQueueLength=1
  wires:
  Blank Message1/1 -> Bus Assignment1/1
  Bus Assignment1/1 -> Publish1/1
  In1/1 -> Display1/1, Bus Assignment1/2

== matlab function Cognata_Amp_Tobi_Split/Subsystem/Median Mental Load ==
  data: HR input; y output; Ratio input; eye input; EyeCondition input
function y = fcn(HR, Ratio, eye, EyeCondition)

if EyeCondition == 0
    vac = [HR Ratio eye];
    y = median(vac);
else 
    vac = [HR Ratio];
    y = median(vac);

end

== matlab function Cognata_Amp_Tobi_Split/Test Components/Filter For smoth RATIO/MATLAB Function2 ==
  data: u input; y output
function y = fcn(u)
    if isnan(u)
        y = 1.0;
    else 
        y=u;
    end
end

== matlab function Cognata_Amp_Tobi_Split/Distance ==
  data: u input; y output
function y = fcn(u)
%#codegen

y = (u*10)+10;

== matlab function Cognata_Amp_Tobi_Split/Test Components/Filter Smoth EYE/Mental load alguritom EYE ==
  data: u input; y output
function y = fcn(u)

y= probability_of_metal_load_EYE(u);

end

== matlab function Cognata_Amp_Tobi_Split/Test Components/Filter For smoth RATIO/Mental load alguritom EEG1 ==
  data: u input; y output
function y = fcn(u)

y= probability_of_metal_load_EEG(u);

end

== matlab function Cognata_Amp_Tobi_Split/Test Components/Filter For smoth RATIO/MATLAB Function4 ==
  data: u input; y output
function y = fcn(u)
%#codegen

y = (u*10)+10;

== matlab function Cognata_Amp_Tobi_Split/Test Components/Filter Smoth EYE/Filter of Nan value ==
  data: u input; y output
function y = fcn(u)

avg = mean(u);

y = avg;

== matlab function Cognata_Amp_Tobi_Split/Test Components/Filter Smoth EYE/MATLAB Function3 ==
  data: u input; y output
function y = fcn(u)
%#codegen

y = (u*10)+10;

== matlab function Cognata_Amp_Tobi_Split/Distance, ==
  data: u input; y output
function y = fcn(u)
%#codegen

y = (u*10)+10;

== matlab function Cognata_Amp_Tobi_Split/Mental load alguritom EYE ==
  data: u input; y output
function y = fcn(u)

y= probability_of_metal_load_EYE(u);

end

== matlab function Cognata_Amp_Tobi_Split/Distance.. ==
  data: u input; y output
function y = fcn(u)
%#codegen

y = (u*10)+10;

== matlab function Cognata_Amp_Tobi_Split/Mental load alguritom GSR ==
  data: u input; y output
function y = fcn(u)

y= probability_of_metal_load_GSR(u);

end

== matlab function Cognata_Amp_Tobi_Split/Distance... ==
  data: u input; y output
function y = fcn(u)
%#codegen

y = (u*10)+10;

== matlab function Cognata_Amp_Tobi_Split/PC timer ==
  data: z output
function z = fcn()
eml.extrinsic('clock'); 
t = [0,0,0,0,0,0];
t = clock;
k = t(1,4:6);
z = k';
end

== matlab function Cognata_Amp_Tobi_Split/Adaptive Component - Time//HR//Distance /Check Mental Load Based on Cordentants ==
  data: Long input; Lat input; y output; Avrage_Menta_Load input
function y = fcn(Long, Lat, Avrage_Menta_Load)
%#codegen

%y = 0;% function output

%if  (30.0 < data )&&(data < 30.1)

decision_time=60.0;
if (decision_time < simulation_time )&&(decision_time+0.1 > simulation_time)% && (Mental_Load < 0.5)    
    
y = 1.0; % SEND MESSAGE

else
    
y = 0.0; % DONT SEND MESSAGE   

end

== matlab function Cognata_Amp_Tobi_Split/Adaptive Component - Time//HR//Distance /Check Mental Load Based on Time ==
  data: Mental_Load input; simulation_time input; y output
function y = fcn(Mental_Load, simulation_time)
%#codegen

%y = 0;% function output

%if  (30.0 < data )&&(data < 30.1)

decision_time=60.0;
if (decision_time < simulation_time )&&(decision_time+0.1 > simulation_time)% && (Mental_Load < 0.5)    
    
y = 1.0; % SEND MESSAGE

else
    
y = 0.0; % DONT SEND MESSAGE   

end

== matlab function Cognata_Amp_Tobi_Split/Mental load alguritom HR ==
  data: u input; y output
function y = fcn(u)

y= probability_of_mental_load_HR(u);

end

== matlab function Cognata_Amp_Tobi_Split/Test Components/Addaptive Component - Distance/MATLAB Function ==
  data: Long1 input; Lat1 input; y output
function y = fcn(Long1, Lat1)
%#codegen

Stop_latitude_Point = 0.0;
Stop_longitude_Point = 0.0;

%y = 0;% function output
Distance_Between_Two_Cordinants_km = deg2km(distance(Long1,Lat1,48.17946869101,11.5851688385))
%if  (30.0 < data )&&(data < 30.1)


if (Distance_Between_Two_Cordinants_km < 0.050)% && (Mental_Load < 0.5)    
    
y = 1.0; % SEND MESSAGE

else
    
y = 0.0; % DONT SEND MESSAGE   

end

== matlab function Cognata_Amp_Tobi_Split/Mental load alguritom EEG  ==
  data: u input; y output
function y = fcn(u)

y= probability_of_metal_load_EEG(u);

end

== matlab function Cognata_Amp_Tobi_Split/Test Components/Filter/Filter HR ==
  data: HR input; y output
function y = fcn(HR)

    
    if HR >= 105.0
     y = 105.0;
    elseif HR <= 94.0 
     y = 94.0;
    else
    y =HR;
    end

   
end

== matlab function Cognata_Amp_Tobi_Split/Test Components/Sigmuid Plot ==
  data: u input; g output
function g = fcn(u)

u = int16(u);

u = (u * 997) + 1.0;

u = int16(u);

x = linspace(-10, 10 ,1000); % vector of x

y = 1 ./ (1 + exp(-x));

% Set the range of x-values
% xlim([-10, 10]);  % range of ציר X


% Plot the function
% figure('MenuBar', 'none', 'ToolBar', 'none');
% fig = figure('Position', [50, 50, 100, 100]);
plot(x, y, 'color', 'red');
hold on


h = plot(x, y, 'o', 'MarkerIndices', u); 
% pause(0.44);
set(h, 'MarkerIndices', []);


g = u;

== matlab function Cognata_Amp_Tobi_Split/Test Components/Filter/Mental load alguritom HR1 ==
  data: u input; y output
function y = fcn(u)

y= probability_of_mental_howrkload(u);

end

== matlab function Cognata_Amp_Tobi_Split/Distance. ==
  data: u input; y output
function y = fcn(u)
%#codegen

y = (u*10)+10;

== matlab function Cognata_Amp_Tobi_Split/Test Components/Filter/Filter Ratio ==
  data: Ratio input; y output
function y = fcn(Ratio)

    
    if Ratio >= -0.125
     y = -0.125;
    elseif Ratio <= -0.0474 
     y = -0.0474;
    else
    y =Ratio;
    end

   
end

== matlab function Cognata_Amp_Tobi_Split/Test Components/Filter/Mental load alguritom EEG1 ==
  data: u input; y output
function y = fcn(u)

y= probability_of_metal_load_EEG(u);

end
